simulink model "digital_twin_control"  (R2023b)
settings: Solver=VariableStepAuto  StartTime=0.0  StopTime=inf  RelTol=1e-3  AbsTol=1e-3  EnableMultiTasking=on
values from neighbouring files (symbols this model uses):
  deltaT = 0.001    [enviroment.m]
  ground = struct()    [enviroment.m]
  robot_conversions = struct()    [joints.m]
  robot_frame = struct()    [enviroment.m]
  robot_joints = struct()    [joints.m]
  robot_weights = struct()    [inertias.m]
  s = tf('s')    [joints.m]
undefined symbols (not defined in the file or in its folder): fractalcoef, LF, X, Y, Z
libraries: sm_lib x101, nesl_utility x29, cstblocks x24, simulink x12, simulink_extras x12, instrumentseriallib x3, mspsensorlib x1
(part 5 of 6)

== system digital_twin_control/Digital Twin (Pavlov Mini)/Back Left Leg/Servomotor + Driver (Hip Joint Y Axis)/Servomotor ==
  PWM Reference : Inport
  Neutral Position (degrees) : Inport  Port=2
  DC to Rad : Subsystem
  Degrees to Radians : simulink_extras/Transformations/Degrees to Radians
  LTI System : cstblocks/LTI System  sys=robot_tf.bessel_filter  IC=[]  PadeOrder=0
  LTI System1 : cstblocks/LTI System  sys=robot_tf.physical_tf  IC=[]  PadeOrder=0
  PS-Simulink Converter : nesl_utility/PS-Simulink Converter  PhysicalDomain=network_engine_domain  SubClassName=ps_output  LeftPortType=input  RightPortType=output  PseudoPeriodic=off  Frequencies=[]  VectorFormat=inherit  Unit=inherit  AffineConversion=off
  Physical Limits : Saturate  UpperLimit=deg2rad(robot_joints.q2_offset+robot_joints.q_limits(2))  LowerLimit=deg2rad(robot_joints.q2_offset+robot_joints.q_limits(1))
  Plus : Sum
  Plus1 : Sum  Inputs=+-
  Servomotor : sm_lib/Joints/Revolute Joint  JointMode=Normal  SenseConstraintForce=off  SenseConstraintForceX=off  SenseConstraintForceY=off  SenseConstraintForceZ=off  SenseConstraintTorque=off  SenseConstraintTorqueX=off  SenseConstraintTorqueY=off  SenseConstraintTorqueZ=off  SenseTotalForce=off  SenseTotalForceX=off  SenseTotalForceY=off  SenseTotalForceZ=off  SenseTotalTorque=off  SenseTotalTorqueX=off  SenseTotalTorqueY=off  SenseTotalTorqueZ=off  CompositeWrenchDir=FollowerOnBase  CompositeWrenchFrame=BaseFrame  EquilibriumPosition=0  EquilibriumPositionUnits=rad  SpringStiffness=0  SpringStiffnessUnits=N*m/deg  DampingCoefficient=0  DampingCoefficientUnits=N*m/(deg/s)  TorqueActuationMode=ComputedTorque  MotionActuationMode=InputMotion  SensePosition=on  SenseVelocity=off  SenseAcceleration=off  SenseTorqueForce=off  SenseLowerLimitTorqueForce=off  SenseUpperLimitTorqueForce=off  LowerLimitSpecify=on  LowerLimitBound=robot_joints.q_limits(1)  LowerLimitBoundUnits=deg  LowerLimitStiffness=1e4  LowerLimitStiffnessUnits=N*m/deg  LowerLimitDamping=10  LowerLimitDampingUnits=N*m/(deg/s)  LowerLimitTransitionRegionWidth=0.1  LowerLimitTransitionRegionWidthUnits=deg  UpperLimitSpecify=on  UpperLimitBound=robot_joints.q_limits(2)  UpperLimitBoundUnits=deg  UpperLimitStiffness=1e4  UpperLimitStiffnessUnits=N*m/deg  UpperLimitDamping=10  UpperLimitDampingUnits=N*m/(deg/s)  UpperLimitTransitionRegionWidth=0.1  UpperLimitTransitionRegionWidthUnits=deg  PositionTargetSpecify=off  PositionTargetPriority=High  PositionTargetValue=0  PositionTargetValueUnits=deg  VelocityTargetSpecify=off  VelocityTargetPriority=High  VelocityTargetValue=0  VelocityTargetValueUnits=deg/s
  Simulink-PS Converter : nesl_utility/Simulink-PS Converter  PhysicalDomain=network_engine_domain  SubClassName=ps_input  LeftPortType=input  RightPortType=output  PseudoPeriodic=off  Frequencies=[]  NoiseDistribution=none  NoiseParameters=[]  Unit=1  AffineConversion=off  FilteringAndDerivatives=filter  SimscapeFilterOrder=2  InputFilterTimeConstant=0.001  UdotUserProvided=0
  Physical Art 1 : PMIOPort  Side=Right
  Physical Art 2 : PMIOPort  Port=2  Side=Right
  Servo Position (rad) : Outport
  wires:
  PWM Reference/1 -> LTI System/1
  LTI System/1 -> LTI System1/1
  LTI System1/1 -> DC to Rad/1(DC (0 -->1))  "DC after physical aproximation"
  Neutral Position (degrees)/1 -> Degrees to Radians/1
  DC to Rad/1(Position (rad)) -> Plus/1  "Position (rad)"
  Plus/1 -> Physical Limits/1  "Position (rad)"
  Degrees to Radians/1 -> Plus1/2, Plus/2
  PS-Simulink Converter/1 -> Plus1/1
  Plus1/1 -> Servo Position (rad)/1
  Physical Limits/1 -> Simulink-PS Converter/1
  connections:
  PS-Simulink Converter/LConn1 -- Servomotor/RConn2
  Physical Art 2/RConn1 -- Servomotor/RConn1
  Servomotor/LConn1 -- Physical Art 1/RConn1
  Servomotor/LConn2 -- Simulink-PS Converter/RConn1

== system digital_twin_control/Digital Twin (Pavlov Mini)/Back Right Leg/Right Leg Without Hip/Servomotor + Driver (Knee Joint Y Axis) ==
  Reference (degrees) : Inport
  Neutral Position (degrees) : Inport  Port=2
  PCA9685 (Aproximation for current Project) : Subsystem
  Servomotor : Subsystem
      settings: PortSchema="{\"entries\":[{\"content\":{\"sides\":[{\"content\":{\"connectorIds\":[\"In1\",\"In2\"]},\"type\":\"ConnectorPlacement.EquallySpacedRectSide\",\"uuid\":\"eeff66d3-7cb0-4fe9-90b5-92935711e170\"},{\"content\":{\"connectorIds\":[\"Out1\"],\"side\":\"RIGHT\"},\"type\":\"ConnectorPlacement.EquallySpacedRectSide\",\"uuid\":\"4c1729b3-3224-4ed4-9eed-359312bd5e7e\"},{\"content\":{\"side\":\"TOP\"},\"type\":\"ConnectorPlacement.EquallySpacedRectSide\",\"uuid\":\"ee6ed6e9-0c82-482d-bf53-5898b89012ab\"},{\"content\":{\"connectorIds\":[\"RConn1\",\"RConn2\"],\"side\":\"BOTTOM\"},\"type\":\"ConnectorPlacement.EquallySpacedRectSide\",\"uuid\":\"6da00c0c-ced6-4450-8de1-d587d7c692e9\"}]},\"type\":\"ConnectorPlacement.EquallySpacedConnector\",\"uuid\":\"38b9234f-cec7-4245-8a78-4426dc0791bf\"}],\"packageUris\":[\"http://schema.mathworks.com/mf0/Connector/R2020b\"],\"version\":\"1.0\"}"
  Physical Art 1 : PMIOPort  Side=Right
  Physical Art 2 : PMIOPort  Port=2  Side=Right
  Servo Position (rad) : Outport
  wires:
  PCA9685 (Aproximation for current Project)/1(PWM Output) -> Servomotor/1(PWM Reference)
  Neutral Position (degrees)/1 -> Servomotor/2(Neutral Position (degrees))
  Reference (degrees)/1 -> PCA9685 (Aproximation for current Project)/1(Reference (degrees))
  Servomotor/1(Servo Position (rad)) -> Servo Position (rad)/1
  connections:
  Servomotor/RConn1 -- Physical Art 1/RConn1
  Physical Art 2/RConn1 -- Servomotor/RConn2

== system digital_twin_control/Digital Twin (Pavlov Mini)/Back Right Leg/Servomotor + Driver (Hip Joint X Axis)/PCA9685 (Aproximation for current Project) ==
  Reference (degrees) : Inport
  Bias : Bias  Bias=robot_conversions.steps_offset  SaturateOnIntegerOverflow=off
  Gain : Gain  Gain=robot_conversions.steps_to_degrees
  Gain1 : Gain  Gain=robot_conversions.degress_to_DC
  PWM : simulink/Discontinuities/PWM  DisableCoverage=on  Period=0.02  InitialDelay=0  DisallowZeroDutyCycle=off  RunAtFixedTimeIntervals=off  SampleTime=0.01
  PWM Output : Outport
  wires:
  Gain/1 -> Bias/1
  Bias/1 -> Gain1/1
  Gain1/1 -> PWM/1
  Reference (degrees)/1 -> Gain/1
  PWM/1 -> PWM Output/1

== system digital_twin_control/Digital Twin (Pavlov Mini)/Back Right Leg/Servomotor + Driver (Hip Joint X Axis)/Servomotor ==
  PWM Reference : Inport
  Neutral Position (degrees) : Inport  Port=2
  DC to Rad : Subsystem
  Degrees to Radians : simulink_extras/Transformations/Degrees to Radians
  LTI System : cstblocks/LTI System  sys=robot_tf.bessel_filter  IC=[]  PadeOrder=0
  LTI System1 : cstblocks/LTI System  sys=robot_tf.physical_tf  IC=[]  PadeOrder=0
  PS-Simulink Converter : nesl_utility/PS-Simulink Converter  PhysicalDomain=network_engine_domain  SubClassName=ps_output  LeftPortType=input  RightPortType=output  PseudoPeriodic=off  Frequencies=[]  VectorFormat=inherit  Unit=inherit  AffineConversion=off
  Physical Limits : Saturate  UpperLimit=deg2rad(-robot_joints.q1_offset+robot_joints.q_limits(2))  LowerLimit=deg2rad(-robot_joints.q1_offset+robot_joints.q_limits(1))
  Plus : Sum
  Plus1 : Sum  Inputs=+-
  Servomotor : sm_lib/Joints/Revolute Joint  JointMode=Normal  SenseConstraintForce=off  SenseConstraintForceX=off  SenseConstraintForceY=off  SenseConstraintForceZ=off  SenseConstraintTorque=off  SenseConstraintTorqueX=off  SenseConstraintTorqueY=off  SenseConstraintTorqueZ=off  SenseTotalForce=off  SenseTotalForceX=off  SenseTotalForceY=off  SenseTotalForceZ=off  SenseTotalTorque=off  SenseTotalTorqueX=off  SenseTotalTorqueY=off  SenseTotalTorqueZ=off  CompositeWrenchDir=FollowerOnBase  CompositeWrenchFrame=BaseFrame  EquilibriumPosition=0  EquilibriumPositionUnits=rad  SpringStiffness=0  SpringStiffnessUnits=N*m/deg  DampingCoefficient=0  DampingCoefficientUnits=N*m/(deg/s)  TorqueActuationMode=ComputedTorque  MotionActuationMode=InputMotion  SensePosition=on  SenseVelocity=off  SenseAcceleration=off  SenseTorqueForce=off  SenseLowerLimitTorqueForce=off  SenseUpperLimitTorqueForce=off  LowerLimitSpecify=on  LowerLimitBound=robot_joints.q_limits(1)-robot_joints.q1_offset  LowerLimitBoundUnits=deg  LowerLimitStiffness=1e4  LowerLimitStiffnessUnits=N*m/deg  LowerLimitDamping=10  LowerLimitDampingUnits=N*m/(deg/s)  LowerLimitTransitionRegionWidth=0.1  LowerLimitTransitionRegionWidthUnits=deg  UpperLimitSpecify=on  UpperLimitBound=robot_joints.q_limits(2)-robot_joints.q1_offset  UpperLimitBoundUnits=deg  UpperLimitStiffness=1e4  UpperLimitStiffnessUnits=N*m/deg  UpperLimitDamping=10  UpperLimitDampingUnits=N*m/(deg/s)  UpperLimitTransitionRegionWidth=0.1  UpperLimitTransitionRegionWidthUnits=deg  PositionTargetSpecify=off  PositionTargetPriority=High  PositionTargetValue=0  PositionTargetValueUnits=deg  VelocityTargetSpecify=off  VelocityTargetPriority=High  VelocityTargetValue=0  VelocityTargetValueUnits=deg/s
  Simulink-PS Converter : nesl_utility/Simulink-PS Converter  PhysicalDomain=network_engine_domain  SubClassName=ps_input  LeftPortType=input  RightPortType=output  PseudoPeriodic=off  Frequencies=[]  NoiseDistribution=none  NoiseParameters=[]  Unit=1  AffineConversion=off  FilteringAndDerivatives=filter  SimscapeFilterOrder=2  InputFilterTimeConstant=0.001  UdotUserProvided=0
  Physical Art 1 : PMIOPort  Side=Right
  Physical Art 2 : PMIOPort  Port=2  Side=Right
  Servo Position (rad) : Outport
  wires:
  PWM Reference/1 -> LTI System/1
  LTI System/1 -> LTI System1/1
  LTI System1/1 -> DC to Rad/1(DC (0 -->1))  "DC after physical aproximation"
  Neutral Position (degrees)/1 -> Degrees to Radians/1
  DC to Rad/1(Position (rad)) -> Plus/1  "Position (rad)"
  Plus/1 -> Physical Limits/1  "Position (rad)"
  Degrees to Radians/1 -> Plus1/2, Plus/2
  PS-Simulink Converter/1 -> Plus1/1
  Plus1/1 -> Servo Position (rad)/1
  Physical Limits/1 -> Simulink-PS Converter/1
  connections:
  PS-Simulink Converter/LConn1 -- Servomotor/RConn2
  Physical Art 2/RConn1 -- Servomotor/RConn1
  Servomotor/LConn1 -- Physical Art 1/RConn1
  Servomotor/LConn2 -- Simulink-PS Converter/RConn1

== system digital_twin_control/Digital Twin (Pavlov Mini)/Back Right Leg/Servomotor + Driver (Hip Joint Y Axis)/PCA9685 (Aproximation for current Project) ==
  Reference (degrees) : Inport
  Bias : Bias  Bias=robot_conversions.steps_offset  SaturateOnIntegerOverflow=off
  Gain : Gain  Gain=robot_conversions.steps_to_degrees
  Gain1 : Gain  Gain=robot_conversions.degress_to_DC
  PWM : simulink/Discontinuities/PWM  DisableCoverage=on  Period=0.02  InitialDelay=0  DisallowZeroDutyCycle=off  RunAtFixedTimeIntervals=off  SampleTime=0.01
  PWM Output : Outport
  wires:
  Gain/1 -> Bias/1
  Bias/1 -> Gain1/1
  Gain1/1 -> PWM/1
  Reference (degrees)/1 -> Gain/1
  PWM/1 -> PWM Output/1

== system digital_twin_control/Digital Twin (Pavlov Mini)/Back Right Leg/Servomotor + Driver (Hip Joint Y Axis)/Servomotor ==
  PWM Reference : Inport
  Neutral Position (degrees) : Inport  Port=2
  DC to Rad : Subsystem
  Degrees to Radians : simulink_extras/Transformations/Degrees to Radians
  LTI System : cstblocks/LTI System  sys=robot_tf.bessel_filter  IC=[]  PadeOrder=0
  LTI System1 : cstblocks/LTI System  sys=robot_tf.physical_tf  IC=[]  PadeOrder=0
  PS-Simulink Converter : nesl_utility/PS-Simulink Converter  PhysicalDomain=network_engine_domain  SubClassName=ps_output  LeftPortType=input  RightPortType=output  PseudoPeriodic=off  Frequencies=[]  VectorFormat=inherit  Unit=inherit  AffineConversion=off
  Physical Limits : Saturate  UpperLimit=deg2rad(-robot_joints.q2_offset+robot_joints.q_limits(2))  LowerLimit=deg2rad(-robot_joints.q2_offset+robot_joints.q_limits(1))
  Plus : Sum
  Plus1 : Sum  Inputs=+-
  Servomotor : sm_lib/Joints/Revolute Joint  JointMode=Normal  SenseConstraintForce=off  SenseConstraintForceX=off  SenseConstraintForceY=off  SenseConstraintForceZ=off  SenseConstraintTorque=off  SenseConstraintTorqueX=off  SenseConstraintTorqueY=off  SenseConstraintTorqueZ=off  SenseTotalForce=off  SenseTotalForceX=off  SenseTotalForceY=off  SenseTotalForceZ=off  SenseTotalTorque=off  SenseTotalTorqueX=off  SenseTotalTorqueY=off  SenseTotalTorqueZ=off  CompositeWrenchDir=FollowerOnBase  CompositeWrenchFrame=BaseFrame  EquilibriumPosition=0  EquilibriumPositionUnits=rad  SpringStiffness=0  SpringStiffnessUnits=N*m/deg  DampingCoefficient=0  DampingCoefficientUnits=N*m/(deg/s)  TorqueActuationMode=ComputedTorque  MotionActuationMode=InputMotion  SensePosition=on  SenseVelocity=off  SenseAcceleration=off  SenseTorqueForce=off  SenseLowerLimitTorqueForce=off  SenseUpperLimitTorqueForce=off  LowerLimitSpecify=on  LowerLimitBound=robot_joints.q_limits(1)-robot_joints.q2_offset  LowerLimitBoundUnits=deg  LowerLimitStiffness=1e4  LowerLimitStiffnessUnits=N*m/deg  LowerLimitDamping=10  LowerLimitDampingUnits=N*m/(deg/s)  LowerLimitTransitionRegionWidth=0.1  LowerLimitTransitionRegionWidthUnits=deg  UpperLimitSpecify=on  UpperLimitBound=robot_joints.q_limits(2)-robot_joints.q2_offset  UpperLimitBoundUnits=deg  UpperLimitStiffness=1e4  UpperLimitStiffnessUnits=N*m/deg  UpperLimitDamping=10  UpperLimitDampingUnits=N*m/(deg/s)  UpperLimitTransitionRegionWidth=0.1  UpperLimitTransitionRegionWidthUnits=deg  PositionTargetSpecify=off  PositionTargetPriority=High  PositionTargetValue=0  PositionTargetValueUnits=deg  VelocityTargetSpecify=off  VelocityTargetPriority=High  VelocityTargetValue=0  VelocityTargetValueUnits=deg/s
  Simulink-PS Converter : nesl_utility/Simulink-PS Converter  PhysicalDomain=network_engine_domain  SubClassName=ps_input  LeftPortType=input  RightPortType=output  PseudoPeriodic=off  Frequencies=[]  NoiseDistribution=none  NoiseParameters=[]  Unit=1  AffineConversion=off  FilteringAndDerivatives=filter  SimscapeFilterOrder=2  InputFilterTimeConstant=0.001  UdotUserProvided=0
  Physical Art 1 : PMIOPort  Side=Right
  Physical Art 2 : PMIOPort  Port=2  Side=Right
  Servo Position (rad) : Outport
  wires:
  PWM Reference/1 -> LTI System/1
  LTI System/1 -> LTI System1/1
  LTI System1/1 -> DC to Rad/1(DC (0 -->1))  "DC after physical aproximation"
  Neutral Position (degrees)/1 -> Degrees to Radians/1
  DC to Rad/1(Position (rad)) -> Plus/1  "Position (rad)"
  Plus/1 -> Physical Limits/1  "Position (rad)"
  Degrees to Radians/1 -> Plus1/2, Plus/2
  PS-Simulink Converter/1 -> Plus1/1
  Plus1/1 -> Servo Position (rad)/1
  Physical Limits/1 -> Simulink-PS Converter/1
  connections:
  PS-Simulink Converter/LConn1 -- Servomotor/RConn2
  Physical Art 2/RConn1 -- Servomotor/RConn1
  Servomotor/LConn1 -- Physical Art 1/RConn1
  Servomotor/LConn2 -- Simulink-PS Converter/RConn1

== system digital_twin_control/Digital Twin (Pavlov Mini)/Front Left Leg/Left Leg Without Hip/Servomotor + Driver (Knee Joint Y Axis) ==
  Reference (degrees) : Inport
  Neutral Position (degrees) : Inport  Port=2
  PCA9685 (Aproximation for current Project) : Subsystem
  Servomotor : Subsystem
      settings: PortSchema="{\"entries\":[{\"content\":{\"sides\":[{\"content\":{\"connectorIds\":[\"In1\",\"In2\"]},\"type\":\"ConnectorPlacement.EquallySpacedRectSide\",\"uuid\":\"eeff66d3-7cb0-4fe9-90b5-92935711e170\"},{\"content\":{\"connectorIds\":[\"Out1\"],\"side\":\"RIGHT\"},\"type\":\"ConnectorPlacement.EquallySpacedRectSide\",\"uuid\":\"4c1729b3-3224-4ed4-9eed-359312bd5e7e\"},{\"content\":{\"side\":\"TOP\"},\"type\":\"ConnectorPlacement.EquallySpacedRectSide\",\"uuid\":\"ee6ed6e9-0c82-482d-bf53-5898b89012ab\"},{\"content\":{\"connectorIds\":[\"RConn1\",\"RConn2\"],\"side\":\"BOTTOM\"},\"type\":\"ConnectorPlacement.EquallySpacedRectSide\",\"uuid\":\"6da00c0c-ced6-4450-8de1-d587d7c692e9\"}]},\"type\":\"ConnectorPlacement.EquallySpacedConnector\",\"uuid\":\"38b9234f-cec7-4245-8a78-4426dc0791bf\"}],\"packageUris\":[\"http://schema.mathworks.com/mf0/Connector/R2020b\"],\"version\":\"1.0\"}"
  Physical Art 1 : PMIOPort  Side=Right
  Physical Art 2 : PMIOPort  Port=2  Side=Right
  Servo Position (rad) : Outport
  wires:
  PCA9685 (Aproximation for current Project)/1(PWM Output) -> Servomotor/1(PWM Reference)
  Neutral Position (degrees)/1 -> Servomotor/2(Neutral Position (degrees))
  Reference (degrees)/1 -> PCA9685 (Aproximation for current Project)/1(Reference (degrees))
  Servomotor/1(Servo Position (rad)) -> Servo Position (rad)/1
  connections:
  Servomotor/RConn1 -- Physical Art 1/RConn1
  Physical Art 2/RConn1 -- Servomotor/RConn2

== system digital_twin_control/Digital Twin (Pavlov Mini)/Front Left Leg/Servomotor + Driver (Hip Joint X Axis)/PCA9685 (Aproximation for current Project) ==
  Reference (degrees) : Inport
  Bias : Bias  Bias=robot_conversions.steps_offset  SaturateOnIntegerOverflow=off
  Gain : Gain  Gain=robot_conversions.steps_to_degrees
  Gain1 : Gain  Gain=robot_conversions.degress_to_DC
  PWM : simulink/Discontinuities/PWM  DisableCoverage=on  Period=0.02  InitialDelay=0  DisallowZeroDutyCycle=off  RunAtFixedTimeIntervals=off  SampleTime=0.01
  PWM Output : Outport
  wires:
  Gain/1 -> Bias/1
  Bias/1 -> Gain1/1
  Gain1/1 -> PWM/1
  Reference (degrees)/1 -> Gain/1
  PWM/1 -> PWM Output/1

== system digital_twin_control/Digital Twin (Pavlov Mini)/Front Left Leg/Servomotor + Driver (Hip Joint X Axis)/Servomotor ==
  PWM Reference : Inport
  Neutral Position (degrees) : Inport  Port=2
  DC to Rad : Subsystem
  Degrees to Radians : simulink_extras/Transformations/Degrees to Radians
  LTI System : cstblocks/LTI System  sys=robot_tf.bessel_filter  IC=[]  PadeOrder=0
  LTI System1 : cstblocks/LTI System  sys=robot_tf.physical_tf  IC=[]  PadeOrder=0
  PS-Simulink Converter : nesl_utility/PS-Simulink Converter  PhysicalDomain=network_engine_domain  SubClassName=ps_output  LeftPortType=input  RightPortType=output  PseudoPeriodic=off  Frequencies=[]  VectorFormat=inherit  Unit=inherit  AffineConversion=off
  Physical Limits : Saturate  UpperLimit=deg2rad(robot_joints.q1_offset+robot_joints.q_limits(2))  LowerLimit=deg2rad(robot_joints.q1_offset+robot_joints.q_limits(1))
  Plus : Sum
  Plus1 : Sum  Inputs=+-
  Servomotor : sm_lib/Joints/Revolute Joint  JointMode=Normal  SenseConstraintForce=off  SenseConstraintForceX=off  SenseConstraintForceY=off  SenseConstraintForceZ=off  SenseConstraintTorque=off  SenseConstraintTorqueX=off  SenseConstraintTorqueY=off  SenseConstraintTorqueZ=off  SenseTotalForce=off  SenseTotalForceX=off  SenseTotalForceY=off  SenseTotalForceZ=off  SenseTotalTorque=off  SenseTotalTorqueX=off  SenseTotalTorqueY=off  SenseTotalTorqueZ=off  CompositeWrenchDir=FollowerOnBase  CompositeWrenchFrame=BaseFrame  EquilibriumPosition=0  EquilibriumPositionUnits=rad  SpringStiffness=0  SpringStiffnessUnits=N*m/deg  DampingCoefficient=0  DampingCoefficientUnits=N*m/(deg/s)  TorqueActuationMode=ComputedTorque  MotionActuationMode=InputMotion  SensePosition=on  SenseVelocity=off  SenseAcceleration=off  SenseTorqueForce=off  SenseLowerLimitTorqueForce=off  SenseUpperLimitTorqueForce=off  LowerLimitSpecify=off  LowerLimitBound=robot_joints.q_limits(1)+robot_joints.q1_offset  LowerLimitBoundUnits=deg  LowerLimitStiffness=1e4  LowerLimitStiffnessUnits=N*m/deg  LowerLimitDamping=10  LowerLimitDampingUnits=N*m/(deg/s)  LowerLimitTransitionRegionWidth=0.1  LowerLimitTransitionRegionWidthUnits=deg  UpperLimitSpecify=off  UpperLimitBound=robot_joints.q_limits(2)+robot_joints.q1_offset  UpperLimitBoundUnits=deg  UpperLimitStiffness=1e4  UpperLimitStiffnessUnits=N*m/deg  UpperLimitDamping=10  UpperLimitDampingUnits=N*m/(deg/s)  UpperLimitTransitionRegionWidth=0.1  UpperLimitTransitionRegionWidthUnits=deg  PositionTargetSpecify=off  PositionTargetPriority=High  PositionTargetValue=0  PositionTargetValueUnits=deg  VelocityTargetSpecify=off  VelocityTargetPriority=High  VelocityTargetValue=0  VelocityTargetValueUnits=deg/s
  Simulink-PS Converter : nesl_utility/Simulink-PS Converter  PhysicalDomain=network_engine_domain  SubClassName=ps_input  LeftPortType=input  RightPortType=output  PseudoPeriodic=off  Frequencies=[]  NoiseDistribution=none  NoiseParameters=[]  Unit=1  AffineConversion=off  FilteringAndDerivatives=filter  SimscapeFilterOrder=2  InputFilterTimeConstant=0.001  UdotUserProvided=0
  Physical Art 1 : PMIOPort  Side=Right
  Physical Art 2 : PMIOPort  Port=2  Side=Right
  Servo Position (rad) : Outport
  wires:
  PWM Reference/1 -> LTI System/1
  LTI System/1 -> LTI System1/1
  LTI System1/1 -> DC to Rad/1(DC (0 -->1))  "DC after physical aproximation"
  Neutral Position (degrees)/1 -> Degrees to Radians/1
  DC to Rad/1(Position (rad)) -> Plus/1  "Position (rad)"
  Plus/1 -> Physical Limits/1  "Position (rad)"
  Degrees to Radians/1 -> Plus1/2, Plus/2
  PS-Simulink Converter/1 -> Plus1/1
  Plus1/1 -> Servo Position (rad)/1
  Physical Limits/1 -> Simulink-PS Converter/1
  connections:
  PS-Simulink Converter/LConn1 -- Servomotor/RConn2
  Physical Art 2/RConn1 -- Servomotor/RConn1
  Servomotor/LConn1 -- Physical Art 1/RConn1
  Servomotor/LConn2 -- Simulink-PS Converter/RConn1

== system digital_twin_control/Digital Twin (Pavlov Mini)/Front Left Leg/Servomotor + Driver (Hip Joint Y Axis)/PCA9685 (Aproximation for current Project) ==
  Reference (degrees) : Inport
  Bias : Bias  Bias=robot_conversions.steps_offset  SaturateOnIntegerOverflow=off
  Gain : Gain  Gain=robot_conversions.steps_to_degrees
  Gain1 : Gain  Gain=robot_conversions.degress_to_DC
  PWM : simulink/Discontinuities/PWM  DisableCoverage=on  Period=0.02  InitialDelay=0  DisallowZeroDutyCycle=off  RunAtFixedTimeIntervals=off  SampleTime=0.01
  PWM Output : Outport
  wires:
  Gain/1 -> Bias/1
  Bias/1 -> Gain1/1
  Gain1/1 -> PWM/1
  Reference (degrees)/1 -> Gain/1
  PWM/1 -> PWM Output/1

== system digital_twin_control/Digital Twin (Pavlov Mini)/Front Left Leg/Servomotor + Driver (Hip Joint Y Axis)/Servomotor ==
  PWM Reference : Inport
  Neutral Position (degrees) : Inport  Port=2
  DC to Rad : Subsystem
  Degrees to Radians : simulink_extras/Transformations/Degrees to Radians
  LTI System : cstblocks/LTI System  sys=robot_tf.bessel_filter  IC=[]  PadeOrder=0
  LTI System1 : cstblocks/LTI System  sys=robot_tf.physical_tf  IC=[]  PadeOrder=0
  PS-Simulink Converter : nesl_utility/PS-Simulink Converter  PhysicalDomain=network_engine_domain  SubClassName=ps_output  LeftPortType=input  RightPortType=output  PseudoPeriodic=off  Frequencies=[]  VectorFormat=inherit  Unit=inherit  AffineConversion=off
  Physical Limits : Saturate  UpperLimit=deg2rad(robot_joints.q2_offset+robot_joints.q_limits(2))  LowerLimit=deg2rad(robot_joints.q2_offset+robot_joints.q_limits(1))
  Plus : Sum
  Plus1 : Sum  Inputs=+-
  Servomotor : sm_lib/Joints/Revolute Joint  JointMode=Normal  SenseConstraintForce=off  SenseConstraintForceX=off  SenseConstraintForceY=off  SenseConstraintForceZ=off  SenseConstraintTorque=off  SenseConstraintTorqueX=off  SenseConstraintTorqueY=off  SenseConstraintTorqueZ=off  SenseTotalForce=off  SenseTotalForceX=off  SenseTotalForceY=off  SenseTotalForceZ=off  SenseTotalTorque=off  SenseTotalTorqueX=off  SenseTotalTorqueY=off  SenseTotalTorqueZ=off  CompositeWrenchDir=FollowerOnBase  CompositeWrenchFrame=BaseFrame  EquilibriumPosition=0  EquilibriumPositionUnits=rad  SpringStiffness=0  SpringStiffnessUnits=N*m/deg  DampingCoefficient=0  DampingCoefficientUnits=N*m/(deg/s)  TorqueActuationMode=ComputedTorque  MotionActuationMode=InputMotion  SensePosition=on  SenseVelocity=off  SenseAcceleration=off  SenseTorqueForce=off  SenseLowerLimitTorqueForce=off  SenseUpperLimitTorqueForce=off  LowerLimitSpecify=off  LowerLimitBound=robot_joints.q_limits(1)+robot_joints.q2_offset  LowerLimitBoundUnits=deg  LowerLimitStiffness=1e4  LowerLimitStiffnessUnits=N*m/deg  LowerLimitDamping=10  LowerLimitDampingUnits=N*m/(deg/s)  LowerLimitTransitionRegionWidth=0.1  LowerLimitTransitionRegionWidthUnits=deg  UpperLimitSpecify=off  UpperLimitBound=robot_joints.q_limits(2)+robot_joints.q2_offset  UpperLimitBoundUnits=deg  UpperLimitStiffness=1e4  UpperLimitStiffnessUnits=N*m/deg  UpperLimitDamping=10  UpperLimitDampingUnits=N*m/(deg/s)  UpperLimitTransitionRegionWidth=0.1  UpperLimitTransitionRegionWidthUnits=deg  PositionTargetSpecify=off  PositionTargetPriority=High  PositionTargetValue=0  PositionTargetValueUnits=deg  VelocityTargetSpecify=off  VelocityTargetPriority=High  VelocityTargetValue=0  VelocityTargetValueUnits=deg/s
  Simulink-PS Converter : nesl_utility/Simulink-PS Converter  PhysicalDomain=network_engine_domain  SubClassName=ps_input  LeftPortType=input  RightPortType=output  PseudoPeriodic=off  Frequencies=[]  NoiseDistribution=none  NoiseParameters=[]  Unit=1  AffineConversion=off  FilteringAndDerivatives=filter  SimscapeFilterOrder=2  InputFilterTimeConstant=0.001  UdotUserProvided=0
  Physical Art 1 : PMIOPort  Side=Right
  Physical Art 2 : PMIOPort  Port=2  Side=Right
  Servo Position (rad) : Outport
  wires:
  PWM Reference/1 -> LTI System/1
  LTI System/1 -> LTI System1/1
  LTI System1/1 -> DC to Rad/1(DC (0 -->1))  "DC after physical aproximation"
  Neutral Position (degrees)/1 -> Degrees to Radians/1
  DC to Rad/1(Position (rad)) -> Plus/1  "Position (rad)"
  Plus/1 -> Physical Limits/1  "Position (rad)"
  Degrees to Radians/1 -> Plus1/2, Plus/2
  PS-Simulink Converter/1 -> Plus1/1
  Plus1/1 -> Servo Position (rad)/1
  Physical Limits/1 -> Simulink-PS Converter/1
  connections:
  PS-Simulink Converter/LConn1 -- Servomotor/RConn2
  Physical Art 2/RConn1 -- Servomotor/RConn1
  Servomotor/LConn1 -- Physical Art 1/RConn1
  Servomotor/LConn2 -- Simulink-PS Converter/RConn1

== system digital_twin_control/Digital Twin (Pavlov Mini)/Front Right Leg/Right Leg Without Hip/Servomotor + Driver (Knee Joint Y Axis) ==
  Reference (degrees) : Inport
  Neutral Position (degrees) : Inport  Port=2
  PCA9685 (Aproximation for current Project) : Subsystem
  Servomotor : Subsystem
      settings: PortSchema="{\"entries\":[{\"content\":{\"sides\":[{\"content\":{\"connectorIds\":[\"In1\",\"In2\"]},\"type\":\"ConnectorPlacement.EquallySpacedRectSide\",\"uuid\":\"eeff66d3-7cb0-4fe9-90b5-92935711e170\"},{\"content\":{\"connectorIds\":[\"Out1\"],\"side\":\"RIGHT\"},\"type\":\"ConnectorPlacement.EquallySpacedRectSide\",\"uuid\":\"4c1729b3-3224-4ed4-9eed-359312bd5e7e\"},{\"content\":{\"side\":\"TOP\"},\"type\":\"ConnectorPlacement.EquallySpacedRectSide\",\"uuid\":\"ee6ed6e9-0c82-482d-bf53-5898b89012ab\"},{\"content\":{\"connectorIds\":[\"RConn1\",\"RConn2\"],\"side\":\"BOTTOM\"},\"type\":\"ConnectorPlacement.EquallySpacedRectSide\",\"uuid\":\"6da00c0c-ced6-4450-8de1-d587d7c692e9\"}]},\"type\":\"ConnectorPlacement.EquallySpacedConnector\",\"uuid\":\"38b9234f-cec7-4245-8a78-4426dc0791bf\"}],\"packageUris\":[\"http://schema.mathworks.com/mf0/Connector/R2020b\"],\"version\":\"1.0\"}"
  Physical Art 1 : PMIOPort  Side=Right
  Physical Art 2 : PMIOPort  Port=2  Side=Right
  Servo Position (rad) : Outport
  wires:
  PCA9685 (Aproximation for current Project)/1(PWM Output) -> Servomotor/1(PWM Reference)
  Neutral Position (degrees)/1 -> Servomotor/2(Neutral Position (degrees))
  Reference (degrees)/1 -> PCA9685 (Aproximation for current Project)/1(Reference (degrees))
  Servomotor/1(Servo Position (rad)) -> Servo Position (rad)/1
  connections:
  Servomotor/RConn1 -- Physical Art 1/RConn1
  Physical Art 2/RConn1 -- Servomotor/RConn2

== system digital_twin_control/Digital Twin (Pavlov Mini)/Front Right Leg/Servomotor + Driver (Hip Joint X Axis)/PCA9685 (Aproximation for current Project) ==
  Reference (degrees) : Inport
  Bias : Bias  Bias=robot_conversions.steps_offset  SaturateOnIntegerOverflow=off
  Gain : Gain  Gain=robot_conversions.steps_to_degrees
  Gain1 : Gain  Gain=robot_conversions.degress_to_DC
  PWM : simulink/Discontinuities/PWM  DisableCoverage=on  Period=0.02  InitialDelay=0  DisallowZeroDutyCycle=off  RunAtFixedTimeIntervals=off  SampleTime=0.01
  PWM Output : Outport
  wires:
  Gain/1 -> Bias/1
  Bias/1 -> Gain1/1
  Gain1/1 -> PWM/1
  Reference (degrees)/1 -> Gain/1
  PWM/1 -> PWM Output/1

== system digital_twin_control/Digital Twin (Pavlov Mini)/Front Right Leg/Servomotor + Driver (Hip Joint X Axis)/Servomotor ==
  PWM Reference : Inport
  Neutral Position (degrees) : Inport  Port=2
  DC to Rad : Subsystem
  Degrees to Radians : simulink_extras/Transformations/Degrees to Radians
  LTI System : cstblocks/LTI System  sys=robot_tf.bessel_filter  IC=[]  PadeOrder=0
  LTI System1 : cstblocks/LTI System  sys=robot_tf.physical_tf  IC=[]  PadeOrder=0
  PS-Simulink Converter : nesl_utility/PS-Simulink Converter  PhysicalDomain=network_engine_domain  SubClassName=ps_output  LeftPortType=input  RightPortType=output  PseudoPeriodic=off  Frequencies=[]  VectorFormat=inherit  Unit=inherit  AffineConversion=off
  Physical Limits : Saturate  UpperLimit=deg2rad(-robot_joints.q1_offset+robot_joints.q_limits(2))  LowerLimit=deg2rad(-robot_joints.q1_offset+robot_joints.q_limits(1))
  Plus : Sum
  Plus1 : Sum  Inputs=+-
  Servomotor : sm_lib/Joints/Revolute Joint  JointMode=Normal  SenseConstraintForce=off  SenseConstraintForceX=off  SenseConstraintForceY=off  SenseConstraintForceZ=off  SenseConstraintTorque=off  SenseConstraintTorqueX=off  SenseConstraintTorqueY=off  SenseConstraintTorqueZ=off  SenseTotalForce=off  SenseTotalForceX=off  SenseTotalForceY=off  SenseTotalForceZ=off  SenseTotalTorque=off  SenseTotalTorqueX=off  SenseTotalTorqueY=off  SenseTotalTorqueZ=off  CompositeWrenchDir=FollowerOnBase  CompositeWrenchFrame=BaseFrame  EquilibriumPosition=0  EquilibriumPositionUnits=rad  SpringStiffness=0  SpringStiffnessUnits=N*m/deg  DampingCoefficient=0  DampingCoefficientUnits=N*m/(deg/s)  TorqueActuationMode=ComputedTorque  MotionActuationMode=InputMotion  SensePosition=on  SenseVelocity=off  SenseAcceleration=off  SenseTorqueForce=off  SenseLowerLimitTorqueForce=off  SenseUpperLimitTorqueForce=off  LowerLimitSpecify=on  LowerLimitBound=robot_joints.q_limits(1)  LowerLimitBoundUnits=deg  LowerLimitStiffness=1e4  LowerLimitStiffnessUnits=N*m/deg  LowerLimitDamping=10  LowerLimitDampingUnits=N*m/(deg/s)  LowerLimitTransitionRegionWidth=0.1  LowerLimitTransitionRegionWidthUnits=deg  UpperLimitSpecify=on  UpperLimitBound=robot_joints.q_limits(2)  UpperLimitBoundUnits=deg  UpperLimitStiffness=1e4  UpperLimitStiffnessUnits=N*m/deg  UpperLimitDamping=10  UpperLimitDampingUnits=N*m/(deg/s)  UpperLimitTransitionRegionWidth=0.1  UpperLimitTransitionRegionWidthUnits=deg  PositionTargetSpecify=off  PositionTargetPriority=High  PositionTargetValue=0  PositionTargetValueUnits=deg  VelocityTargetSpecify=off  VelocityTargetPriority=High  VelocityTargetValue=0  VelocityTargetValueUnits=deg/s
  Simulink-PS Converter : nesl_utility/Simulink-PS Converter  PhysicalDomain=network_engine_domain  SubClassName=ps_input  LeftPortType=input  RightPortType=output  PseudoPeriodic=off  Frequencies=[]  NoiseDistribution=none  NoiseParameters=[]  Unit=1  AffineConversion=off  FilteringAndDerivatives=filter  SimscapeFilterOrder=2  InputFilterTimeConstant=0.001  UdotUserProvided=0
  Physical Art 1 : PMIOPort  Side=Right
  Physical Art 2 : PMIOPort  Port=2  Side=Right
  Servo Position (rad) : Outport
  wires:
  PWM Reference/1 -> LTI System/1
  LTI System/1 -> LTI System1/1
  LTI System1/1 -> DC to Rad/1(DC (0 -->1))  "DC after physical aproximation"
  Neutral Position (degrees)/1 -> Degrees to Radians/1
  DC to Rad/1(Position (rad)) -> Plus/1  "Position (rad)"
  Plus/1 -> Physical Limits/1  "Position (rad)"
  Degrees to Radians/1 -> Plus1/2, Plus/2
  PS-Simulink Converter/1 -> Plus1/1
  Plus1/1 -> Servo Position (rad)/1
  Physical Limits/1 -> Simulink-PS Converter/1
  connections:
  PS-Simulink Converter/LConn1 -- Servomotor/RConn2
  Physical Art 2/RConn1 -- Servomotor/RConn1
  Servomotor/LConn1 -- Physical Art 1/RConn1
  Servomotor/LConn2 -- Simulink-PS Converter/RConn1

== system digital_twin_control/Digital Twin (Pavlov Mini)/Front Right Leg/Servomotor + Driver (Hip Joint Y Axis)/PCA9685 (Aproximation for current Project) ==
  Reference (degrees) : Inport
  Bias : Bias  Bias=robot_conversions.steps_offset  SaturateOnIntegerOverflow=off
  Gain : Gain  Gain=robot_conversions.steps_to_degrees
  Gain1 : Gain  Gain=robot_conversions.degress_to_DC
  PWM : simulink/Discontinuities/PWM  DisableCoverage=on  Period=0.02  InitialDelay=0  DisallowZeroDutyCycle=off  RunAtFixedTimeIntervals=off  SampleTime=0.01
  PWM Output : Outport
  wires:
  Gain/1 -> Bias/1
  Bias/1 -> Gain1/1
  Gain1/1 -> PWM/1
  Reference (degrees)/1 -> Gain/1
  PWM/1 -> PWM Output/1

== system digital_twin_control/Digital Twin (Pavlov Mini)/Front Right Leg/Servomotor + Driver (Hip Joint Y Axis)/Servomotor ==
  PWM Reference : Inport
  Neutral Position (degrees) : Inport  Port=2
  DC to Rad : Subsystem
  Degrees to Radians : simulink_extras/Transformations/Degrees to Radians
  LTI System : cstblocks/LTI System  sys=robot_tf.bessel_filter  IC=[]  PadeOrder=0
  LTI System1 : cstblocks/LTI System  sys=robot_tf.physical_tf  IC=[]  PadeOrder=0
  PS-Simulink Converter : nesl_utility/PS-Simulink Converter  PhysicalDomain=network_engine_domain  SubClassName=ps_output  LeftPortType=input  RightPortType=output  PseudoPeriodic=off  Frequencies=[]  VectorFormat=inherit  Unit=inherit  AffineConversion=off
  Physical Limits : Saturate  UpperLimit=deg2rad(-robot_joints.q2_offset+robot_joints.q_limits(2))  LowerLimit=deg2rad(-robot_joints.q2_offset+robot_joints.q_limits(1))
  Plus : Sum
  Plus1 : Sum  Inputs=+-
  Servomotor : sm_lib/Joints/Revolute Joint  JointMode=Normal  SenseConstraintForce=off  SenseConstraintForceX=off  SenseConstraintForceY=off  SenseConstraintForceZ=off  SenseConstraintTorque=off  SenseConstraintTorqueX=off  SenseConstraintTorqueY=off  SenseConstraintTorqueZ=off  SenseTotalForce=off  SenseTotalForceX=off  SenseTotalForceY=off  SenseTotalForceZ=off  SenseTotalTorque=off  SenseTotalTorqueX=off  SenseTotalTorqueY=off  SenseTotalTorqueZ=off  CompositeWrenchDir=FollowerOnBase  CompositeWrenchFrame=BaseFrame  EquilibriumPosition=0  EquilibriumPositionUnits=rad  SpringStiffness=0  SpringStiffnessUnits=N*m/deg  DampingCoefficient=0  DampingCoefficientUnits=N*m/(deg/s)  TorqueActuationMode=ComputedTorque  MotionActuationMode=InputMotion  SensePosition=on  SenseVelocity=off  SenseAcceleration=off  SenseTorqueForce=off  SenseLowerLimitTorqueForce=off  SenseUpperLimitTorqueForce=off  LowerLimitSpecify=on  LowerLimitBound=robot_joints.q_limits(1)  LowerLimitBoundUnits=deg  LowerLimitStiffness=1e4  LowerLimitStiffnessUnits=N*m/deg  LowerLimitDamping=10  LowerLimitDampingUnits=N*m/(deg/s)  LowerLimitTransitionRegionWidth=0.1  LowerLimitTransitionRegionWidthUnits=deg  UpperLimitSpecify=on  UpperLimitBound=robot_joints.q_limits(2)  UpperLimitBoundUnits=deg  UpperLimitStiffness=1e4  UpperLimitStiffnessUnits=N*m/deg  UpperLimitDamping=10  UpperLimitDampingUnits=N*m/(deg/s)  UpperLimitTransitionRegionWidth=0.1  UpperLimitTransitionRegionWidthUnits=deg  PositionTargetSpecify=off  PositionTargetPriority=High  PositionTargetValue=0  PositionTargetValueUnits=deg  VelocityTargetSpecify=off  VelocityTargetPriority=High  VelocityTargetValue=0  VelocityTargetValueUnits=deg/s
  Simulink-PS Converter : nesl_utility/Simulink-PS Converter  PhysicalDomain=network_engine_domain  SubClassName=ps_input  LeftPortType=input  RightPortType=output  PseudoPeriodic=off  Frequencies=[]  NoiseDistribution=none  NoiseParameters=[]  Unit=1  AffineConversion=off  FilteringAndDerivatives=filter  SimscapeFilterOrder=2  InputFilterTimeConstant=0.001  UdotUserProvided=0
  Physical Art 1 : PMIOPort  Side=Right
  Physical Art 2 : PMIOPort  Port=2  Side=Right
  Servo Position (rad) : Outport
  wires:
  PWM Reference/1 -> LTI System/1
  LTI System/1 -> LTI System1/1
  LTI System1/1 -> DC to Rad/1(DC (0 -->1))  "DC after physical aproximation"
  Neutral Position (degrees)/1 -> Degrees to Radians/1
  DC to Rad/1(Position (rad)) -> Plus/1  "Position (rad)"
  Plus/1 -> Physical Limits/1  "Position (rad)"
  Degrees to Radians/1 -> Plus1/2, Plus/2
  PS-Simulink Converter/1 -> Plus1/1
  Plus1/1 -> Servo Position (rad)/1
  Physical Limits/1 -> Simulink-PS Converter/1
  connections:
  PS-Simulink Converter/LConn1 -- Servomotor/RConn2
  Physical Art 2/RConn1 -- Servomotor/RConn1
  Servomotor/LConn1 -- Physical Art 1/RConn1
  Servomotor/LConn2 -- Simulink-PS Converter/RConn1

== system digital_twin_control/Digital Twin (Pavlov Mini)/Back Left Leg/Left Leg Without Hip/Servomotor + Driver (Knee Joint Y Axis)/PCA9685 (Aproximation for current Project) ==
  Reference (degrees) : Inport
  Bias : Bias  Bias=robot_conversions.steps_offset  SaturateOnIntegerOverflow=off
  Gain : Gain  Gain=robot_conversions.steps_to_degrees
  Gain1 : Gain  Gain=robot_conversions.degress_to_DC
  PWM : simulink/Discontinuities/PWM  DisableCoverage=on  Period=0.02  InitialDelay=0  DisallowZeroDutyCycle=off  RunAtFixedTimeIntervals=off  SampleTime=0.01
  PWM Output : Outport
  wires:
  Gain/1 -> Bias/1
  Bias/1 -> Gain1/1
  Gain1/1 -> PWM/1
  Reference (degrees)/1 -> Gain/1
  PWM/1 -> PWM Output/1

== system digital_twin_control/Digital Twin (Pavlov Mini)/Back Left Leg/Left Leg Without Hip/Servomotor + Driver (Knee Joint Y Axis)/Servomotor ==
  PWM Reference : Inport
  Neutral Position (degrees) : Inport  Port=2
  DC to Rad : Subsystem
  Degrees to Radians : simulink_extras/Transformations/Degrees to Radians
  LTI System : cstblocks/LTI System  sys=robot_tf.bessel_filter  IC=[]  PadeOrder=0
  LTI System1 : cstblocks/LTI System  sys=robot_tf.physical_tf  IC=[]  PadeOrder=0
  PS-Simulink Converter : nesl_utility/PS-Simulink Converter  PhysicalDomain=network_engine_domain  SubClassName=ps_output  LeftPortType=input  RightPortType=output  PseudoPeriodic=off  Frequencies=[]  VectorFormat=inherit  Unit=inherit  AffineConversion=off
  Physical Limits : Saturate  UpperLimit=deg2rad(robot_joints.q3_offset+robot_joints.q_limits(2))  LowerLimit=deg2rad(robot_joints.q3_offset+robot_joints.q_limits(1))
  Plus : Sum
  Plus1 : Sum  Inputs=+-
  Servomotor : sm_lib/Joints/Revolute Joint  JointMode=Normal  SenseConstraintForce=off  SenseConstraintForceX=off  SenseConstraintForceY=off  SenseConstraintForceZ=off  SenseConstraintTorque=off  SenseConstraintTorqueX=off  SenseConstraintTorqueY=off  SenseConstraintTorqueZ=off  SenseTotalForce=off  SenseTotalForceX=off  SenseTotalForceY=off  SenseTotalForceZ=off  SenseTotalTorque=off  SenseTotalTorqueX=off  SenseTotalTorqueY=off  SenseTotalTorqueZ=off  CompositeWrenchDir=FollowerOnBase  CompositeWrenchFrame=BaseFrame  EquilibriumPosition=0  EquilibriumPositionUnits=rad  SpringStiffness=0  SpringStiffnessUnits=N*m/deg  DampingCoefficient=0  DampingCoefficientUnits=N*m/(deg/s)  TorqueActuationMode=ComputedTorque  MotionActuationMode=InputMotion  SensePosition=on  SenseVelocity=off  SenseAcceleration=off  SenseTorqueForce=off  SenseLowerLimitTorqueForce=off  SenseUpperLimitTorqueForce=off  LowerLimitSpecify=on  LowerLimitBound=robot_joints.q_limits(1)  LowerLimitBoundUnits=deg  LowerLimitStiffness=1e4  LowerLimitStiffnessUnits=N*m/deg  LowerLimitDamping=10  LowerLimitDampingUnits=N*m/(deg/s)  LowerLimitTransitionRegionWidth=0.1  LowerLimitTransitionRegionWidthUnits=deg  UpperLimitSpecify=on  UpperLimitBound=robot_joints.q_limits(2)  UpperLimitBoundUnits=deg  UpperLimitStiffness=1e4  UpperLimitStiffnessUnits=N*m/deg  UpperLimitDamping=10  UpperLimitDampingUnits=N*m/(deg/s)  UpperLimitTransitionRegionWidth=0.1  UpperLimitTransitionRegionWidthUnits=deg  PositionTargetSpecify=off  PositionTargetPriority=High  PositionTargetValue=0  PositionTargetValueUnits=deg  VelocityTargetSpecify=off  VelocityTargetPriority=High  VelocityTargetValue=0  VelocityTargetValueUnits=deg/s
  Simulink-PS Converter : nesl_utility/Simulink-PS Converter  PhysicalDomain=network_engine_domain  SubClassName=ps_input  LeftPortType=input  RightPortType=output  PseudoPeriodic=off  Frequencies=[]  NoiseDistribution=none  NoiseParameters=[]  Unit=1  AffineConversion=off  FilteringAndDerivatives=filter  SimscapeFilterOrder=2  InputFilterTimeConstant=0.001  UdotUserProvided=0
  Physical Art 1 : PMIOPort  Side=Right
  Physical Art 2 : PMIOPort  Port=2  Side=Right
  Servo Position (rad) : Outport
  wires:
  PWM Reference/1 -> LTI System/1
  LTI System/1 -> LTI System1/1
  LTI System1/1 -> DC to Rad/1(DC (0 -->1))  "DC after physical aproximation"
  Neutral Position (degrees)/1 -> Degrees to Radians/1
  DC to Rad/1(Position (rad)) -> Plus/1  "Position (rad)"
  Plus/1 -> Physical Limits/1  "Position (rad)"
  Degrees to Radians/1 -> Plus1/2, Plus/2
  PS-Simulink Converter/1 -> Plus1/1
  Plus1/1 -> Servo Position (rad)/1
  Physical Limits/1 -> Simulink-PS Converter/1
  connections:
  PS-Simulink Converter/LConn1 -- Servomotor/RConn2
  Physical Art 2/RConn1 -- Servomotor/RConn1
  Servomotor/LConn1 -- Physical Art 1/RConn1
  Servomotor/LConn2 -- Simulink-PS Converter/RConn1

== system digital_twin_control/Digital Twin (Pavlov Mini)/Back Left Leg/Servomotor + Driver (Hip Joint X Axis)/Servomotor/DC to Rad ==
  DC (0 -->1) : Inport
  Bias2 : Bias  Bias=robot_conversions.DC_offset  SaturateOnIntegerOverflow=off
  Gain2 : Gain  Gain=robot_conversions.DC_to_rad
  Position (rad) : Outport
  wires:
  DC (0 -->1)/1 -> Bias2/1
  Bias2/1 -> Gain2/1
  Gain2/1 -> Position (rad)/1

== system digital_twin_control/Digital Twin (Pavlov Mini)/Back Left Leg/Servomotor + Driver (Hip Joint Y Axis)/Servomotor/DC to Rad ==
  DC (0 -->1) : Inport
  Bias2 : Bias  Bias=robot_conversions.DC_offset  SaturateOnIntegerOverflow=off
  Gain2 : Gain  Gain=robot_conversions.DC_to_rad
  Position (rad) : Outport
  wires:
  DC (0 -->1)/1 -> Bias2/1
  Bias2/1 -> Gain2/1
  Gain2/1 -> Position (rad)/1

== system digital_twin_control/Digital Twin (Pavlov Mini)/Back Right Leg/Right Leg Without Hip/Servomotor + Driver (Knee Joint Y Axis)/PCA9685 (Aproximation for current Project) ==
  Reference (degrees) : Inport
  Bias : Bias  Bias=robot_conversions.steps_offset  SaturateOnIntegerOverflow=off
  Gain : Gain  Gain=robot_conversions.steps_to_degrees
  Gain1 : Gain  Gain=robot_conversions.degress_to_DC
  PWM : simulink/Discontinuities/PWM  DisableCoverage=on  Period=0.02  InitialDelay=0  DisallowZeroDutyCycle=off  RunAtFixedTimeIntervals=off  SampleTime=0.01
  PWM Output : Outport
  wires:
  Gain/1 -> Bias/1
  Bias/1 -> Gain1/1
  Gain1/1 -> PWM/1
  Reference (degrees)/1 -> Gain/1
  PWM/1 -> PWM Output/1

== system digital_twin_control/Digital Twin (Pavlov Mini)/Back Right Leg/Right Leg Without Hip/Servomotor + Driver (Knee Joint Y Axis)/Servomotor ==
  PWM Reference : Inport
  Neutral Position (degrees) : Inport  Port=2
  DC to Rad : Subsystem
  Degrees to Radians : simulink_extras/Transformations/Degrees to Radians
  LTI System : cstblocks/LTI System  sys=robot_tf.bessel_filter  IC=[]  PadeOrder=0
  LTI System1 : cstblocks/LTI System  sys=robot_tf.physical_tf  IC=[]  PadeOrder=0
  PS-Simulink Converter : nesl_utility/PS-Simulink Converter  PhysicalDomain=network_engine_domain  SubClassName=ps_output  LeftPortType=input  RightPortType=output  PseudoPeriodic=off  Frequencies=[]  VectorFormat=inherit  Unit=inherit  AffineConversion=off
  Physical Limits : Saturate  UpperLimit=deg2rad(-robot_joints.q3_offset+robot_joints.q_limits(2))  LowerLimit=deg2rad(-robot_joints.q3_offset+robot_joints.q_limits(1))
  Plus : Sum
  Plus1 : Sum  Inputs=+-
  Servomotor : sm_lib/Joints/Revolute Joint  JointMode=Normal  SenseConstraintForce=off  SenseConstraintForceX=off  SenseConstraintForceY=off  SenseConstraintForceZ=off  SenseConstraintTorque=off  SenseConstraintTorqueX=off  SenseConstraintTorqueY=off  SenseConstraintTorqueZ=off  SenseTotalForce=off  SenseTotalForceX=off  SenseTotalForceY=off  SenseTotalForceZ=off  SenseTotalTorque=off  SenseTotalTorqueX=off  SenseTotalTorqueY=off  SenseTotalTorqueZ=off  CompositeWrenchDir=FollowerOnBase  CompositeWrenchFrame=BaseFrame  EquilibriumPosition=0  EquilibriumPositionUnits=rad  SpringStiffness=0  SpringStiffnessUnits=N*m/deg  DampingCoefficient=0  DampingCoefficientUnits=N*m/(deg/s)  TorqueActuationMode=ComputedTorque  MotionActuationMode=InputMotion  SensePosition=on  SenseVelocity=off  SenseAcceleration=off  SenseTorqueForce=off  SenseLowerLimitTorqueForce=off  SenseUpperLimitTorqueForce=off  LowerLimitSpecify=on  LowerLimitBound=robot_joints.q_limits(1)-robot_joints.q3_offset  LowerLimitBoundUnits=deg  LowerLimitStiffness=1e4  LowerLimitStiffnessUnits=N*m/deg  LowerLimitDamping=10  LowerLimitDampingUnits=N*m/(deg/s)  LowerLimitTransitionRegionWidth=0.1  LowerLimitTransitionRegionWidthUnits=deg  UpperLimitSpecify=on  UpperLimitBound=robot_joints.q_limits(2)-robot_joints.q3_offset  UpperLimitBoundUnits=deg  UpperLimitStiffness=1e4  UpperLimitStiffnessUnits=N*m/deg  UpperLimitDamping=10  UpperLimitDampingUnits=N*m/(deg/s)  UpperLimitTransitionRegionWidth=0.1  UpperLimitTransitionRegionWidthUnits=deg  PositionTargetSpecify=off  PositionTargetPriority=High  PositionTargetValue=0  PositionTargetValueUnits=deg  VelocityTargetSpecify=off  VelocityTargetPriority=High  VelocityTargetValue=0  VelocityTargetValueUnits=deg/s
  Simulink-PS Converter : nesl_utility/Simulink-PS Converter  PhysicalDomain=network_engine_domain  SubClassName=ps_input  LeftPortType=input  RightPortType=output  PseudoPeriodic=off  Frequencies=[]  NoiseDistribution=none  NoiseParameters=[]  Unit=1  AffineConversion=off  FilteringAndDerivatives=filter  SimscapeFilterOrder=2  InputFilterTimeConstant=0.001  UdotUserProvided=0
  Physical Art 1 : PMIOPort  Side=Right
  Physical Art 2 : PMIOPort  Port=2  Side=Right
  Servo Position (rad) : Outport
  wires:
  PWM Reference/1 -> LTI System/1
  LTI System/1 -> LTI System1/1
  LTI System1/1 -> DC to Rad/1(DC (0 -->1))  "DC after physical aproximation"
  Neutral Position (degrees)/1 -> Degrees to Radians/1
  DC to Rad/1(Position (rad)) -> Plus/1  "Position (rad)"
  Plus/1 -> Physical Limits/1  "Position (rad)"
  Degrees to Radians/1 -> Plus1/2, Plus/2
  PS-Simulink Converter/1 -> Plus1/1
  Plus1/1 -> Servo Position (rad)/1
  Physical Limits/1 -> Simulink-PS Converter/1
  connections:
  PS-Simulink Converter/LConn1 -- Servomotor/RConn2
  Physical Art 2/RConn1 -- Servomotor/RConn1
  Servomotor/LConn1 -- Physical Art 1/RConn1
  Servomotor/LConn2 -- Simulink-PS Converter/RConn1

== system digital_twin_control/Digital Twin (Pavlov Mini)/Back Right Leg/Servomotor + Driver (Hip Joint X Axis)/Servomotor/DC to Rad ==
  DC (0 -->1) : Inport
  Bias2 : Bias  Bias=robot_conversions.DC_offset  SaturateOnIntegerOverflow=off
  Gain2 : Gain  Gain=robot_conversions.DC_to_rad
  Position (rad) : Outport
  wires:
  DC (0 -->1)/1 -> Bias2/1
  Bias2/1 -> Gain2/1
  Gain2/1 -> Position (rad)/1

== system digital_twin_control/Digital Twin (Pavlov Mini)/Back Right Leg/Servomotor + Driver (Hip Joint Y Axis)/Servomotor/DC to Rad ==
  DC (0 -->1) : Inport
  Bias2 : Bias  Bias=robot_conversions.DC_offset  SaturateOnIntegerOverflow=off
  Gain2 : Gain  Gain=robot_conversions.DC_to_rad
  Position (rad) : Outport
  wires:
  DC (0 -->1)/1 -> Bias2/1
  Bias2/1 -> Gain2/1
  Gain2/1 -> Position (rad)/1

== system digital_twin_control/Digital Twin (Pavlov Mini)/Front Left Leg/Left Leg Without Hip/Servomotor + Driver (Knee Joint Y Axis)/PCA9685 (Aproximation for current Project) ==
  Reference (degrees) : Inport
  Bias : Bias  Bias=robot_conversions.steps_offset  SaturateOnIntegerOverflow=off
  Gain : Gain  Gain=robot_conversions.steps_to_degrees
  Gain1 : Gain  Gain=robot_conversions.degress_to_DC
  PWM : simulink/Discontinuities/PWM  DisableCoverage=on  Period=0.02  InitialDelay=0  DisallowZeroDutyCycle=off  RunAtFixedTimeIntervals=off  SampleTime=0.01
  PWM Output : Outport
  wires:
  Gain/1 -> Bias/1
  Bias/1 -> Gain1/1
  Gain1/1 -> PWM/1
  Reference (degrees)/1 -> Gain/1
  PWM/1 -> PWM Output/1
